simulink model "exact_state_observer_model"  (R2024b)
settings: Solver=FixedStepAuto  StartTime=0.0  StopTime=T_final  FixedStep=dt  MaxStep=1e-2  RelTol=1e-3
values from neighbouring files (symbols this model uses):
  A = [0  1; 0  0]    [data_T_05_tau_1e2.mat]    (also in data_T_2_tau1e3.mat; exact_state_observer.m = input('Specify matrix A (in the form of an n x n matrix): '))
  B = [0 1]    [data_T_05_tau_1e2.mat]    (also in data_T_2_tau1e3.mat; exact_state_observer.m = input('Give matrix B (in the form of an n x 1 matrix): '))
  C = [2 0]    [data_T_05_tau_1e2.mat]    (also in data_T_2_tau1e3.mat; exact_state_observer.m = input('Give matrix C (in the form of a 1 x n matrix): '))
  D = 0    [data_T_05_tau_1e2.mat]    (also in data_T_2_tau1e3.mat; exact_state_observer.m = input('Give final matrix D: '))
settings Model: Creator=Paweł Wiktor  LastModifiedBy=Paweł Wiktor
settings DataIOCC: ReturnWorkspaceOutputs=off

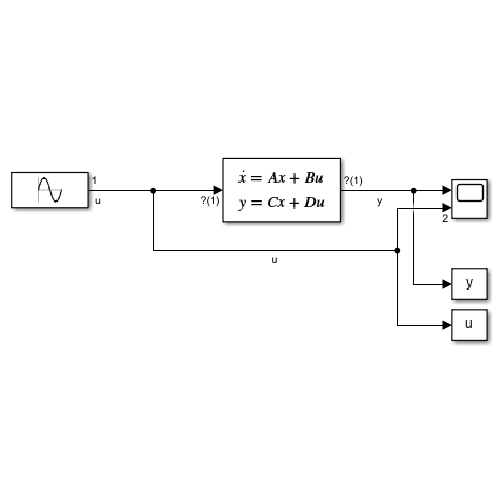
[thumbnail: Simulink's stored preview of the top-level diagram]
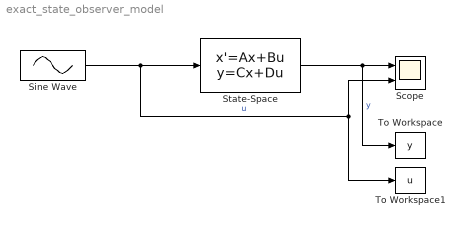
== system exact_state_observer_model ==
  Scope : Scope  NumInputPorts=2
  Sine Wave : Sin  Frequency=2*pi  SampleTime=0
  State-Space : StateSpace  A=A  B=B  C=C  D=D  InitialCondition=0
  To Workspace : ToWorkspace  VariableName=y  SampleTime=-1
  To Workspace1 : ToWorkspace  VariableName=u  SampleTime=-1
  wires:
  State-Space/1 -> To Workspace/1, Scope/1  "y"
  Sine Wave/1 -> State-Space/1, Scope/2, To Workspace1/1  "u"
